simulink model "Inverter_PI"  (R2016a)
settings: Solver=ode23t  StartTime=0.0  StopTime=0.1  FixedStep=t_PWM/10  MaxStep=2e-6  RelTol=2e-4
values from neighbouring files (symbols this model uses):
  Rs = sol(3)    [SolarPanelModel.m]
  t_PWM = 20e-6    (= 2e-05)    [SolarPanelModel.m]
  Vo = 50    [SolarPanelModel.m]
undefined symbols (not defined in the file or in its folder): a, Cdc_inv, Ci, Po, Td, Tzv, Vgrid
libraries: powerlib x7
settings Model: Creator=frede  LastModifiedBy=frede
settings DataIOCC: LimitDataPoints=on  SaveFormat=Array
settings HardwareCC: ProdBitPerPointer=32  ProdLargestAtomicFloat=None  ProdIntDivRoundTo=Undefined  ProdEndianess=Unspecified  ProdWordSize=32  ProdHWDeviceType=32-bit Generic
settings ModelReferenceCC: PropagateSignalLabelsOutOfModel=off
settings ConfigComp: CovModelRefEnable=Off

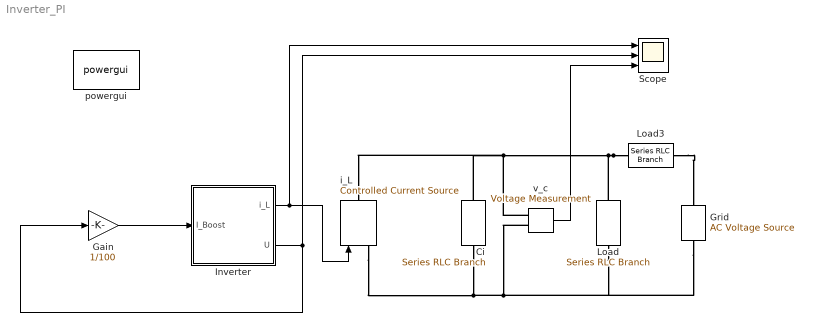
== system Inverter_PI ==
  Ci : powerlib/Elements/Series RLC Branch  LConnTagsString=__new0  RConnTagsString=__new0  BranchType=C  Resistance=Rs  Inductance=1e-3  SetiL0=off  InitialCurrent=0  Capacitance=Ci  Setx0=off  InitialVoltage=0  Measurements=None
  Gain : Gain  Gain=1/100
  Grid : powerlib/Electrical Sources/AC Voltage Source  Amplitude=230*sqrt(2)  Phase=0  Frequency=50  SampleTime=0  Measurements=None  BusType=swing  Pref=10e3  Qref=0  Qmin=-inf  Qmax=+inf
  Inverter : Subsystem
  Load : powerlib/Elements/Series RLC Branch  LConnTagsString=__new0  RConnTagsString=__new0  BranchType=R  Resistance=Vgrid^2/Po  Inductance=1e-3  SetiL0=off  InitialCurrent=0  Capacitance=1e-6  Setx0=off  InitialVoltage=0  Measurements=None
  Load3 : powerlib/Elements/Series RLC Branch  LConnTagsString=__new0  RConnTagsString=__new0  BranchType=R  Resistance=0.001  Inductance=1e-3  SetiL0=off  InitialCurrent=0  Capacitance=1e-6  Setx0=off  InitialVoltage=0  Measurements=None
  Scope : Scope  NumInputPorts=3
  i_L : powerlib/Electrical Sources/Controlled Current Source  Initialize=on  Source_Type=AC  Amplitude=0  Phase=0  Frequency=0  Measurements=None
  powergui : powerlib/powergui  Priority=1  SimulationMode=Discrete  SolverType=Tustin/Backward Euler (TBE)  SampleTime=t_PWM/10  frequency=60  SPID=off  DisableSnubberDevices=off  DisableRonSwitches=off  DisableVfSwitches=off  SwTol=0  DisplayEquations=off  Interpol=off  ExternalGateDelay=off  methode=off  Ts=10  FunctionMessages=off  echomessages=off  HookPort=off  EnableUseOfTLC=off  x0status=blocks  frequencyindice=0  Pbase=100e6  ErrMax=1e-4  Iterations=50  UnitsV=kV  UnitsW=MW  buscounter=0  RestoreLinks=warning  ResistiveCurrentMeasurement=off  Frange=[0:2:500]  Ylog=off  Xlog=on  ShowGrid=off  save=off  variable=ZData  structure=0  ZoomFFT=off  StartTime=0.0  cycles=1  DisplayStyle=1  fundamental=60  FreqAxis=off  MaxFrequency=1000  frequencyindicesteady=1  RmsSteady=1  display=off
  v_c : powerlib/Measurements/Voltage Measurement  PhasorSimulation=off  OutputType=Complex  PSBequivalent=0
  wires:
  Inverter/1(i_L) -> Scope/1, i_L/1
  Inverter/2(U) -> Scope/2, Gain/1
  Gain/1 -> Inverter/1(I_Boost)
  v_c/1 -> Scope/3
  connections:
  i_L/LConn1 -- v_c/LConn2 -- Load/RConn1 -- Grid/LConn1 -- Ci/RConn1
  Load3/RConn1 -- Grid/RConn1
  Load3/LConn1 -- Ci/LConn1 -- i_L/RConn1 -- v_c/LConn1 -- Load/LConn1

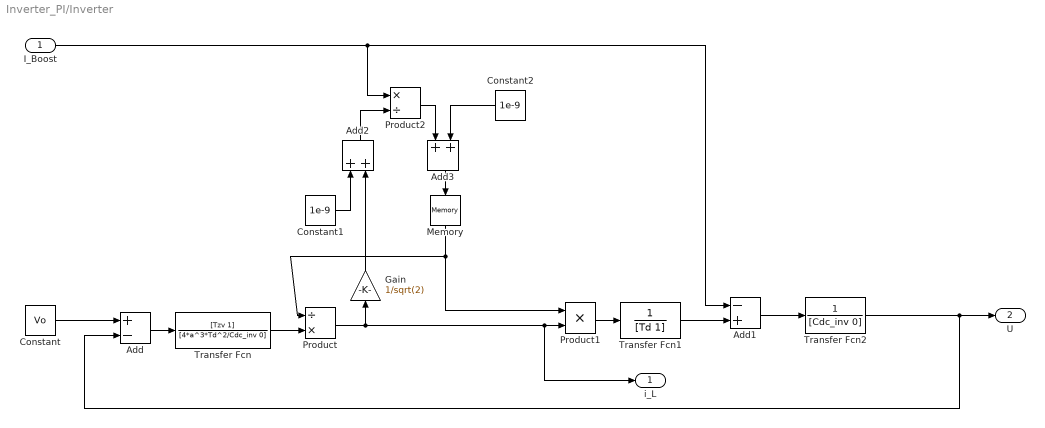
== system Inverter_PI/Inverter ==
  I_Boost : Inport
  Add : Sum  Inputs=+-
  Add1 : Sum  Inputs=-+
  Add2 : Sum
  Add3 : Sum
  Constant : Constant  Value=Vo
  Constant1 : Constant  Value=1e-9
  Constant2 : Constant  Value=1e-9
  Gain : Gain  Gain=1/sqrt(2)
  Memory : Memory  X0=1e-9
  Product : Product  Inputs=/*
  Product1 : Product
  Product2 : Product  Inputs=*/
  Transfer Fcn : TransferFcn  Numerator=[Tzv 1]  Denominator=[4*a^3*Td^2/Cdc_inv 0]
  Transfer Fcn1 : TransferFcn  Denominator=[Td 1]
  Transfer Fcn2 : TransferFcn  Denominator=[Cdc_inv 0]
  i_L : Outport
  U : Outport  Port=2
  wires:
  Constant/1 -> Add/1
  Add/1 -> Transfer Fcn/1
  Transfer Fcn2/1 -> Add/2, U/1
  Transfer Fcn1/1 -> Add1/2
  I_Boost/1 -> Product2/1, Add1/1
  Add1/1 -> Transfer Fcn2/1
  Transfer Fcn/1 -> Product/2
  Product1/1 -> Transfer Fcn1/1
  Product/1 -> Gain/1, i_L/1, Product1/2
  Product2/1 -> Add3/1
  Add3/1 -> Memory/1
  Gain/1 -> Add2/2
  Add2/1 -> Product2/2
  Constant1/1 -> Add2/1
  Constant2/1 -> Add3/2
  Memory/1 -> Product/1, Product1/1
